simulink subsystem "Mk3SerialNeckWrapper"  (R2025a)
settings: Solver=VariableStepAuto  StartTime=0.0  StopTime=10.0  RelTol=1e-3
undefined symbols (not defined in the file): Joint1_B, Joint1_F, Joint2_B, Joint2_F, Joint3_B, Joint3_F, Payload_base_frame, Transmission1_Stage1, Transmission2_Stage1, Transmission3_Stage1, X, Y, Z
libraries: sm_lib x1
settings Model: DataDictionary=neck_mk3.sldd  EnableAccessToBaseWorkspace=off  Creator=upattacini  LastModifiedBy=upattacini
settings RTWCC: GPUComputeCapability=3.5

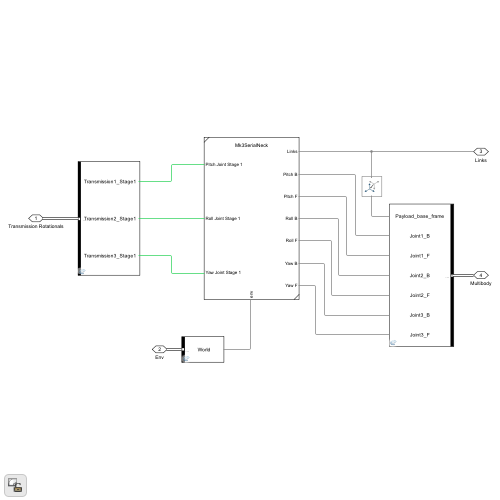
[thumbnail: Simulink's stored preview of the top-level diagram]
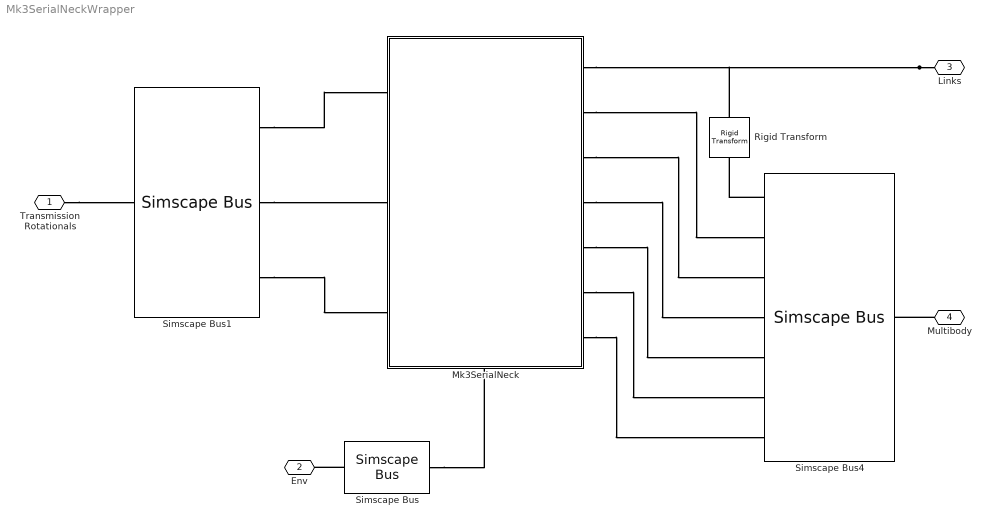
== system Mk3SerialNeckWrapper ==
  Mk3SerialNeck : Subsystem  ReferencedSubsystem=Mk3SerialNeck
      settings: PermitHierarchicalResolution=None  PortSchema="{\"entries\":[{\"content\":{\"sides\":[{\"content\":{\"connectorIds\":[\"LConn1\",\"LConn2\",\"LConn3\"]},\"type\":\"ConnectorPlacement.EquallySpacedRectSide\",\"uuid\":\"4b888494-381c-4272-8abc-8f83eebfec7f\"},{\"content\":{\"connectorIds\":[\"RConn1\",\"RConn2\",\"RConn3\",\"RConn4\",\"RConn5\",\"RConn6\",\"RConn7\"],\"side\":\"RIGHT\"},\"type\":\"ConnectorPlacement.EquallySpacedRectSide\",\"uuid\":\"5e2fb81a-98a3-4540-ad18-4e565f40b72d\"},{\"content\":{\"side\":\"TOP\"},\"type\":\"ConnectorPlacement.EquallySpacedRectSide\",\"uuid\":\"931a4bcf-b447-442d-bbb9-fcef6a7da2eb\"},{\"content\":{\"connectorIds\":[\"RConn8\"],\"side\":\"BOTTOM\"},\"type\":\"ConnectorPlacement.EquallySpacedRectSide\",\"uuid\":\"e5ae3658-dcf6-4f22-bc0e-be12e7cf504d\"}]},\"type\":\"ConnectorPlacement.EquallySpacedConnector\",\"uuid\":\"beb28445-7a73-4fff-b796-4545b9b3a7b7\"}],\"packageUris\":[\"http://schema.mathworks.com/mf0/Connector/R2020b\"],\"version\":\"1.0\"}"
  Rigid Transform : sm_lib/Frames and Transforms/Rigid Transform  RotationMethod=StandardAxis  FollAlignAxisA=+X  BaseAlignAxisA=+Y  FollAlignAxisB=+Y  BaseAlignAxisB=+Z  RotationStandardAxis=-X  RotationAngle=90  RotationAngleUnits=deg  RotationArbitraryAxis=[0 0 1]  RotationSequenceAxes=FollowerAxes  RotationSequence=XYX  RotationSequenceAngles=[0 0 0]  RotationSequenceAnglesUnits=deg  RotationMatrix=[0 1 0; 0 0 1; 1 0 0]  Quaternion=[1 0 0 0]  TranslationMethod=None  TranslationCartesianOffset=[0 0 0]  TranslationCartesianOffsetUnits=m  TranslationStandardAxis=+Z  TranslationStandardOffset=0  TranslationStandardOffsetUnits=m  TranslationROffset=0  TranslationROffsetUnits=m  TranslationThetaOffset=0  TranslationThetaOffsetUnits=deg  TranslationZOffset=0  TranslationZOffsetUnits=m
  Simscape Bus : SimscapeBus  HierarchyStrings=World  ConnectionType=Bus: Physical_Environment
  Simscape Bus1 : SimscapeBus  HierarchyStrings=Transmission1_Stage1;Transmission2_Stage1;Transmission3_Stage1  ConnectionType=Bus: Physical_TransmissionRotationals
  Simscape Bus4 : SimscapeBus  HierarchyStrings=Payload_base_frame;Joint1_B;Joint1_F;Joint2_B;Joint2_F;Joint3_B;Joint3_F  ConnectionType=Bus: Physical_Multibody
  Transmission Rotationals : PMIOPort  Side=Left
  Env : PMIOPort  Port=2  Side=Right
  Links : PMIOPort  Port=3  Side=Right
  Multibody : PMIOPort  Port=4  Side=Right
  connections:
  Links/RConn1 -- Mk3SerialNeck/RConn1 -- Rigid Transform/LConn1
  Simscape Bus/RConn1 -- Env/RConn1
  Transmission Rotationals/RConn1 -- Simscape Bus1/RConn1
  Multibody/RConn1 -- Simscape Bus4/RConn1
  Mk3SerialNeck/RConn2 -- Simscape Bus4/LConn2
  Mk3SerialNeck/RConn3 -- Simscape Bus4/LConn3
  Mk3SerialNeck/RConn4 -- Simscape Bus4/LConn4
  Mk3SerialNeck/RConn5 -- Simscape Bus4/LConn5
  Mk3SerialNeck/RConn6 -- Simscape Bus4/LConn6
  Mk3SerialNeck/RConn7 -- Simscape Bus4/LConn7
  Simscape Bus4/LConn1 -- Rigid Transform/RConn1
  Simscape Bus/LConn1 -- Mk3SerialNeck/RConn8
  Simscape Bus1/LConn2 -- Mk3SerialNeck/LConn2
  Simscape Bus1/LConn1 -- Mk3SerialNeck/LConn1
  Simscape Bus1/LConn3 -- Mk3SerialNeck/LConn3
